simulink model "waterTankBurner"  (R2014b)
settings: Solver=ode1  StartTime=0.0  StopTime=100  FixedStep=0.0001  MaxStep=0.0001  RelTol=1e-3
(part 2 of 4)

== system waterTankBurner/waterTank31 ==
  note: integrator t4
  ON : Inport
  OFF : Inport  Port=2
  INIT y1 : Constant  Value=20
  INIT y3 : Constant  Value=100
  Integrator b{1..4} (4 alike) : DiscreteIntegrator  ExternalReset=either  InitialConditionSource=external  InitialCondition=510  InitialConditionSetting=State (most efficient)  SampleTime=-1
  MATLAB Function : MATLAB Function  Priority=1  TreatAsAtomicUnit=on
  MATLAB Function1 : MATLAB Function  TreatAsAtomicUnit=on
  Multiport Switch : MultiPortSwitch  Inputs=4
  Scope : Scope  NumInputPorts=8
      settings: TickLabels=on  ShowLegends=on  YMin=0~0~0~0~0~0~0~0  YMax=1~1~1~1~1~1~1~1
  q : Memory  X0=1  LinearizeMemory=on
  reset1 : Memory  LinearizeMemory=on
  xx : Memory  LinearizeMemory=on
  x : Outport
  wires:
  INIT y1/1 -> Integrator b1/3
  MATLAB Function1/1(ode1) -> Integrator b1/1
  MATLAB Function/1(qNext) -> q/1  "q_before"
  q/1 -> Multiport Switch/1, MATLAB Function/1(q), Scope/1  "q_after"
  MATLAB Function/2(reset) -> reset1/1
  MATLAB Function1/2(ode2) -> Integrator b2/1
  INIT y3/1 -> Integrator b3/3
  MATLAB Function1/3(ode3) -> Integrator b3/1
  MATLAB Function1/4(ode4) -> Integrator b4/1
  reset1/1 -> Integrator b4/2, Integrator b3/2, Integrator b2/2, Integrator b1/2  "reset_after"
  Integrator b1/1 -> Multiport Switch/2  "integrator t1"
  Integrator b2/1 -> Multiport Switch/3  "integrator t2"
  Integrator b3/1 -> Multiport Switch/4  "integrator t3"
  Integrator b4/1 -> Multiport Switch/5
  OFF/1 -> MATLAB Function/3(OFF)
  ON/1 -> MATLAB Function/2(ON)
  xx/1 -> x/1, Scope/2, Integrator b2/3, Integrator b4/3, MATLAB Function1/1(x), MATLAB Function/4(x)
  Multiport Switch/1 -> xx/1  "x"

== system waterTankBurner/waterTank32 ==
  note: integrator t4
  ON : Inport
  OFF : Inport  Port=2
  INIT y1 : Constant  Value=20
  INIT y3 : Constant  Value=100
  Integrator b{1..4} (4 alike) : DiscreteIntegrator  ExternalReset=either  InitialConditionSource=external  InitialCondition=510  InitialConditionSetting=State (most efficient)  SampleTime=-1
  MATLAB Function : MATLAB Function  Priority=1  TreatAsAtomicUnit=on
  MATLAB Function1 : MATLAB Function  TreatAsAtomicUnit=on
  Multiport Switch : MultiPortSwitch  Inputs=4
  Scope : Scope  NumInputPorts=8
      settings: TickLabels=on  ShowLegends=on  YMin=0~0~0~0~0~0~0~0  YMax=1~1~1~1~1~1~1~1
  q : Memory  X0=1  LinearizeMemory=on
  reset1 : Memory  LinearizeMemory=on
  xx : Memory  LinearizeMemory=on
  x : Outport
  wires:
  INIT y1/1 -> Integrator b1/3
  MATLAB Function1/1(ode1) -> Integrator b1/1
  MATLAB Function/1(qNext) -> q/1  "q_before"
  q/1 -> Multiport Switch/1, MATLAB Function/1(q), Scope/1  "q_after"
  MATLAB Function/2(reset) -> reset1/1
  MATLAB Function1/2(ode2) -> Integrator b2/1
  INIT y3/1 -> Integrator b3/3
  MATLAB Function1/3(ode3) -> Integrator b3/1
  MATLAB Function1/4(ode4) -> Integrator b4/1
  reset1/1 -> Integrator b4/2, Integrator b3/2, Integrator b2/2, Integrator b1/2  "reset_after"
  Integrator b1/1 -> Multiport Switch/2  "integrator t1"
  Integrator b2/1 -> Multiport Switch/3  "integrator t2"
  Integrator b3/1 -> Multiport Switch/4  "integrator t3"
  Integrator b4/1 -> Multiport Switch/5
  OFF/1 -> MATLAB Function/3(OFF)
  ON/1 -> MATLAB Function/2(ON)
  xx/1 -> x/1, Scope/2, Integrator b2/3, Integrator b4/3, MATLAB Function1/1(x), MATLAB Function/4(x)
  Multiport Switch/1 -> xx/1  "x"

== system waterTankBurner/waterTank33 ==
  note: integrator t4
  ON : Inport
  OFF : Inport  Port=2
  INIT y1 : Constant  Value=20
  INIT y3 : Constant  Value=100
  Integrator b{1..4} (4 alike) : DiscreteIntegrator  ExternalReset=either  InitialConditionSource=external  InitialCondition=510  InitialConditionSetting=State (most efficient)  SampleTime=-1
  MATLAB Function : MATLAB Function  Priority=1  TreatAsAtomicUnit=on
  MATLAB Function1 : MATLAB Function  TreatAsAtomicUnit=on
  Multiport Switch : MultiPortSwitch  Inputs=4
  Scope : Scope  NumInputPorts=8
      settings: TickLabels=on  ShowLegends=on  YMin=0~0~0~0~0~0~0~0  YMax=1~1~1~1~1~1~1~1
  q : Memory  X0=1  LinearizeMemory=on
  reset1 : Memory  LinearizeMemory=on
  xx : Memory  LinearizeMemory=on
  x : Outport
  wires:
  INIT y1/1 -> Integrator b1/3
  MATLAB Function1/1(ode1) -> Integrator b1/1
  MATLAB Function/1(qNext) -> q/1  "q_before"
  q/1 -> Multiport Switch/1, MATLAB Function/1(q), Scope/1  "q_after"
  MATLAB Function/2(reset) -> reset1/1
  MATLAB Function1/2(ode2) -> Integrator b2/1
  INIT y3/1 -> Integrator b3/3
  MATLAB Function1/3(ode3) -> Integrator b3/1
  MATLAB Function1/4(ode4) -> Integrator b4/1
  reset1/1 -> Integrator b4/2, Integrator b3/2, Integrator b2/2, Integrator b1/2  "reset_after"
  Integrator b1/1 -> Multiport Switch/2  "integrator t1"
  Integrator b2/1 -> Multiport Switch/3  "integrator t2"
  Integrator b3/1 -> Multiport Switch/4  "integrator t3"
  Integrator b4/1 -> Multiport Switch/5
  OFF/1 -> MATLAB Function/3(OFF)
  ON/1 -> MATLAB Function/2(ON)
  xx/1 -> x/1, Scope/2, Integrator b2/3, Integrator b4/3, MATLAB Function1/1(x), MATLAB Function/4(x)
  Multiport Switch/1 -> xx/1  "x"

== system waterTankBurner/waterTank34 ==
  note: integrator t4
  ON : Inport
  OFF : Inport  Port=2
  INIT y1 : Constant  Value=20
  INIT y3 : Constant  Value=100
  Integrator b{1..4} (4 alike) : DiscreteIntegrator  ExternalReset=either  InitialConditionSource=external  InitialCondition=510  InitialConditionSetting=State (most efficient)  SampleTime=-1
  MATLAB Function : MATLAB Function  Priority=1  TreatAsAtomicUnit=on
  MATLAB Function1 : MATLAB Function  TreatAsAtomicUnit=on
  Multiport Switch : MultiPortSwitch  Inputs=4
  Scope : Scope  NumInputPorts=8
      settings: TickLabels=on  ShowLegends=on  YMin=0~0~0~0~0~0~0~0  YMax=1~1~1~1~1~1~1~1
  q : Memory  X0=1  LinearizeMemory=on
  reset1 : Memory  LinearizeMemory=on
  xx : Memory  LinearizeMemory=on
  x : Outport
  wires:
  INIT y1/1 -> Integrator b1/3
  MATLAB Function1/1(ode1) -> Integrator b1/1
  MATLAB Function/1(qNext) -> q/1  "q_before"
  q/1 -> Multiport Switch/1, MATLAB Function/1(q), Scope/1  "q_after"
  MATLAB Function/2(reset) -> reset1/1
  MATLAB Function1/2(ode2) -> Integrator b2/1
  INIT y3/1 -> Integrator b3/3
  MATLAB Function1/3(ode3) -> Integrator b3/1
  MATLAB Function1/4(ode4) -> Integrator b4/1
  reset1/1 -> Integrator b4/2, Integrator b3/2, Integrator b2/2, Integrator b1/2  "reset_after"
  Integrator b1/1 -> Multiport Switch/2  "integrator t1"
  Integrator b2/1 -> Multiport Switch/3  "integrator t2"
  Integrator b3/1 -> Multiport Switch/4  "integrator t3"
  Integrator b4/1 -> Multiport Switch/5
  OFF/1 -> MATLAB Function/3(OFF)
  ON/1 -> MATLAB Function/2(ON)
  xx/1 -> x/1, Scope/2, Integrator b2/3, Integrator b4/3, MATLAB Function1/1(x), MATLAB Function/4(x)
  Multiport Switch/1 -> xx/1  "x"

== system waterTankBurner/waterTank35 ==
  note: integrator t4
  ON : Inport
  OFF : Inport  Port=2
  INIT y1 : Constant  Value=20
  INIT y3 : Constant  Value=100
  Integrator b{1..4} (4 alike) : DiscreteIntegrator  ExternalReset=either  InitialConditionSource=external  InitialCondition=510  InitialConditionSetting=State (most efficient)  SampleTime=-1
  MATLAB Function : MATLAB Function  Priority=1  TreatAsAtomicUnit=on
  MATLAB Function1 : MATLAB Function  TreatAsAtomicUnit=on
  Multiport Switch : MultiPortSwitch  Inputs=4
  Scope : Scope  NumInputPorts=8
      settings: TickLabels=on  ShowLegends=on  YMin=0~0~0~0~0~0~0~0  YMax=1~1~1~1~1~1~1~1
  q : Memory  X0=1  LinearizeMemory=on
  reset1 : Memory  LinearizeMemory=on
  xx : Memory  LinearizeMemory=on
  x : Outport
  wires:
  INIT y1/1 -> Integrator b1/3
  MATLAB Function1/1(ode1) -> Integrator b1/1
  MATLAB Function/1(qNext) -> q/1  "q_before"
  q/1 -> Multiport Switch/1, MATLAB Function/1(q), Scope/1  "q_after"
  MATLAB Function/2(reset) -> reset1/1
  MATLAB Function1/2(ode2) -> Integrator b2/1
  INIT y3/1 -> Integrator b3/3
  MATLAB Function1/3(ode3) -> Integrator b3/1
  MATLAB Function1/4(ode4) -> Integrator b4/1
  reset1/1 -> Integrator b4/2, Integrator b3/2, Integrator b2/2, Integrator b1/2  "reset_after"
  Integrator b1/1 -> Multiport Switch/2  "integrator t1"
  Integrator b2/1 -> Multiport Switch/3  "integrator t2"
  Integrator b3/1 -> Multiport Switch/4  "integrator t3"
  Integrator b4/1 -> Multiport Switch/5
  OFF/1 -> MATLAB Function/3(OFF)
  ON/1 -> MATLAB Function/2(ON)
  xx/1 -> x/1, Scope/2, Integrator b2/3, Integrator b4/3, MATLAB Function1/1(x), MATLAB Function/4(x)
  Multiport Switch/1 -> xx/1  "x"

== system waterTankBurner/waterTank36 ==
  note: integrator t4
  ON : Inport
  OFF : Inport  Port=2
  INIT y1 : Constant  Value=20
  INIT y3 : Constant  Value=100
  Integrator b{1..4} (4 alike) : DiscreteIntegrator  ExternalReset=either  InitialConditionSource=external  InitialCondition=510  InitialConditionSetting=State (most efficient)  SampleTime=-1
  MATLAB Function : MATLAB Function  Priority=1  TreatAsAtomicUnit=on
  MATLAB Function1 : MATLAB Function  TreatAsAtomicUnit=on
  Multiport Switch : MultiPortSwitch  Inputs=4
  Scope : Scope  NumInputPorts=8
      settings: TickLabels=on  ShowLegends=on  YMin=0~0~0~0~0~0~0~0  YMax=1~1~1~1~1~1~1~1
  q : Memory  X0=1  LinearizeMemory=on
  reset1 : Memory  LinearizeMemory=on
  xx : Memory  LinearizeMemory=on
  x : Outport
  wires:
  INIT y1/1 -> Integrator b1/3
  MATLAB Function1/1(ode1) -> Integrator b1/1
  MATLAB Function/1(qNext) -> q/1  "q_before"
  q/1 -> Multiport Switch/1, MATLAB Function/1(q), Scope/1  "q_after"
  MATLAB Function/2(reset) -> reset1/1
  MATLAB Function1/2(ode2) -> Integrator b2/1
  INIT y3/1 -> Integrator b3/3
  MATLAB Function1/3(ode3) -> Integrator b3/1
  MATLAB Function1/4(ode4) -> Integrator b4/1
  reset1/1 -> Integrator b4/2, Integrator b3/2, Integrator b2/2, Integrator b1/2  "reset_after"
  Integrator b1/1 -> Multiport Switch/2  "integrator t1"
  Integrator b2/1 -> Multiport Switch/3  "integrator t2"
  Integrator b3/1 -> Multiport Switch/4  "integrator t3"
  Integrator b4/1 -> Multiport Switch/5
  OFF/1 -> MATLAB Function/3(OFF)
  ON/1 -> MATLAB Function/2(ON)
  xx/1 -> x/1, Scope/2, Integrator b2/3, Integrator b4/3, MATLAB Function1/1(x), MATLAB Function/4(x)
  Multiport Switch/1 -> xx/1  "x"

== system waterTankBurner/waterTank37 ==
  note: integrator t4
  ON : Inport
  OFF : Inport  Port=2
  INIT y1 : Constant  Value=20
  INIT y3 : Constant  Value=100
  Integrator b{1..4} (4 alike) : DiscreteIntegrator  ExternalReset=either  InitialConditionSource=external  InitialCondition=510  InitialConditionSetting=State (most efficient)  SampleTime=-1
  MATLAB Function : MATLAB Function  Priority=1  TreatAsAtomicUnit=on
  MATLAB Function1 : MATLAB Function  TreatAsAtomicUnit=on
  Multiport Switch : MultiPortSwitch  Inputs=4
  Scope : Scope  NumInputPorts=8
      settings: TickLabels=on  ShowLegends=on  YMin=0~0~0~0~0~0~0~0  YMax=1~1~1~1~1~1~1~1
  q : Memory  X0=1  LinearizeMemory=on
  reset1 : Memory  LinearizeMemory=on
  xx : Memory  LinearizeMemory=on
  x : Outport
  wires:
  INIT y1/1 -> Integrator b1/3
  MATLAB Function1/1(ode1) -> Integrator b1/1
  MATLAB Function/1(qNext) -> q/1  "q_before"
  q/1 -> Multiport Switch/1, MATLAB Function/1(q), Scope/1  "q_after"
  MATLAB Function/2(reset) -> reset1/1
  MATLAB Function1/2(ode2) -> Integrator b2/1
  INIT y3/1 -> Integrator b3/3
  MATLAB Function1/3(ode3) -> Integrator b3/1
  MATLAB Function1/4(ode4) -> Integrator b4/1
  reset1/1 -> Integrator b4/2, Integrator b3/2, Integrator b2/2, Integrator b1/2  "reset_after"
  Integrator b1/1 -> Multiport Switch/2  "integrator t1"
  Integrator b2/1 -> Multiport Switch/3  "integrator t2"
  Integrator b3/1 -> Multiport Switch/4  "integrator t3"
  Integrator b4/1 -> Multiport Switch/5
  OFF/1 -> MATLAB Function/3(OFF)
  ON/1 -> MATLAB Function/2(ON)
  xx/1 -> x/1, Scope/2, Integrator b2/3, Integrator b4/3, MATLAB Function1/1(x), MATLAB Function/4(x)
  Multiport Switch/1 -> xx/1  "x"

== system waterTankBurner/waterTank38 ==
  note: integrator t4
  ON : Inport
  OFF : Inport  Port=2
  INIT y1 : Constant  Value=20
  INIT y3 : Constant  Value=100
  Integrator b{1..4} (4 alike) : DiscreteIntegrator  ExternalReset=either  InitialConditionSource=external  InitialCondition=510  InitialConditionSetting=State (most efficient)  SampleTime=-1
  MATLAB Function : MATLAB Function  Priority=1  TreatAsAtomicUnit=on
  MATLAB Function1 : MATLAB Function  TreatAsAtomicUnit=on
  Multiport Switch : MultiPortSwitch  Inputs=4
  Scope : Scope  NumInputPorts=8
      settings: TickLabels=on  ShowLegends=on  YMin=0~0~0~0~0~0~0~0  YMax=1~1~1~1~1~1~1~1
  q : Memory  X0=1  LinearizeMemory=on
  reset1 : Memory  LinearizeMemory=on
  xx : Memory  LinearizeMemory=on
  x : Outport
  wires:
  INIT y1/1 -> Integrator b1/3
  MATLAB Function1/1(ode1) -> Integrator b1/1
  MATLAB Function/1(qNext) -> q/1  "q_before"
  q/1 -> Multiport Switch/1, MATLAB Function/1(q), Scope/1  "q_after"
  MATLAB Function/2(reset) -> reset1/1
  MATLAB Function1/2(ode2) -> Integrator b2/1
  INIT y3/1 -> Integrator b3/3
  MATLAB Function1/3(ode3) -> Integrator b3/1
  MATLAB Function1/4(ode4) -> Integrator b4/1
  reset1/1 -> Integrator b4/2, Integrator b3/2, Integrator b2/2, Integrator b1/2  "reset_after"
  Integrator b1/1 -> Multiport Switch/2  "integrator t1"
  Integrator b2/1 -> Multiport Switch/3  "integrator t2"
  Integrator b3/1 -> Multiport Switch/4  "integrator t3"
  Integrator b4/1 -> Multiport Switch/5
  OFF/1 -> MATLAB Function/3(OFF)
  ON/1 -> MATLAB Function/2(ON)
  xx/1 -> x/1, Scope/2, Integrator b2/3, Integrator b4/3, MATLAB Function1/1(x), MATLAB Function/4(x)
  Multiport Switch/1 -> xx/1  "x"

== system waterTankBurner/waterTank39 ==
  note: integrator t4
  ON : Inport
  OFF : Inport  Port=2
  INIT y1 : Constant  Value=20
  INIT y3 : Constant  Value=100
  Integrator b{1..4} (4 alike) : DiscreteIntegrator  ExternalReset=either  InitialConditionSource=external  InitialCondition=510  InitialConditionSetting=State (most efficient)  SampleTime=-1
  MATLAB Function : MATLAB Function  Priority=1  TreatAsAtomicUnit=on
  MATLAB Function1 : MATLAB Function  TreatAsAtomicUnit=on
  Multiport Switch : MultiPortSwitch  Inputs=4
  Scope : Scope  NumInputPorts=8
      settings: TickLabels=on  ShowLegends=on  YMin=0~0~0~0~0~0~0~0  YMax=1~1~1~1~1~1~1~1
  q : Memory  X0=1  LinearizeMemory=on
  reset1 : Memory  LinearizeMemory=on
  xx : Memory  LinearizeMemory=on
  x : Outport
  wires:
  INIT y1/1 -> Integrator b1/3
  MATLAB Function1/1(ode1) -> Integrator b1/1
  MATLAB Function/1(qNext) -> q/1  "q_before"
  q/1 -> Multiport Switch/1, MATLAB Function/1(q), Scope/1  "q_after"
  MATLAB Function/2(reset) -> reset1/1
  MATLAB Function1/2(ode2) -> Integrator b2/1
  INIT y3/1 -> Integrator b3/3
  MATLAB Function1/3(ode3) -> Integrator b3/1
  MATLAB Function1/4(ode4) -> Integrator b4/1
  reset1/1 -> Integrator b4/2, Integrator b3/2, Integrator b2/2, Integrator b1/2  "reset_after"
  Integrator b1/1 -> Multiport Switch/2  "integrator t1"
  Integrator b2/1 -> Multiport Switch/3  "integrator t2"
  Integrator b3/1 -> Multiport Switch/4  "integrator t3"
  Integrator b4/1 -> Multiport Switch/5
  OFF/1 -> MATLAB Function/3(OFF)
  ON/1 -> MATLAB Function/2(ON)
  xx/1 -> x/1, Scope/2, Integrator b2/3, Integrator b4/3, MATLAB Function1/1(x), MATLAB Function/4(x)
  Multiport Switch/1 -> xx/1  "x"

== system waterTankBurner/waterTank4 ==
  note: integrator t4
  ON : Inport
  OFF : Inport  Port=2
  INIT y1 : Constant  Value=20
  INIT y3 : Constant  Value=100
  Integrator b{1..4} (4 alike) : DiscreteIntegrator  ExternalReset=either  InitialConditionSource=external  InitialCondition=510  InitialConditionSetting=State (most efficient)  SampleTime=-1
  MATLAB Function : MATLAB Function  Priority=1  TreatAsAtomicUnit=on
  MATLAB Function1 : MATLAB Function  TreatAsAtomicUnit=on
  Multiport Switch : MultiPortSwitch  Inputs=4
  Scope : Scope  NumInputPorts=8
      settings: TickLabels=on  ShowLegends=on  YMin=0~0~0~0~0~0~0~0  YMax=1~1~1~1~1~1~1~1
  q : Memory  X0=1  LinearizeMemory=on
  reset1 : Memory  LinearizeMemory=on
  xx : Memory  LinearizeMemory=on
  x : Outport
  wires:
  INIT y1/1 -> Integrator b1/3
  MATLAB Function1/1(ode1) -> Integrator b1/1
  MATLAB Function/1(qNext) -> q/1  "q_before"
  q/1 -> Multiport Switch/1, MATLAB Function/1(q), Scope/1  "q_after"
  MATLAB Function/2(reset) -> reset1/1
  MATLAB Function1/2(ode2) -> Integrator b2/1
  INIT y3/1 -> Integrator b3/3
  MATLAB Function1/3(ode3) -> Integrator b3/1
  MATLAB Function1/4(ode4) -> Integrator b4/1
  reset1/1 -> Integrator b4/2, Integrator b3/2, Integrator b2/2, Integrator b1/2  "reset_after"
  Integrator b1/1 -> Multiport Switch/2  "integrator t1"
  Integrator b2/1 -> Multiport Switch/3  "integrator t2"
  Integrator b3/1 -> Multiport Switch/4  "integrator t3"
  Integrator b4/1 -> Multiport Switch/5
  OFF/1 -> MATLAB Function/3(OFF)
  ON/1 -> MATLAB Function/2(ON)
  xx/1 -> x/1, Scope/2, Integrator b2/3, Integrator b4/3, MATLAB Function1/1(x), MATLAB Function/4(x)
  Multiport Switch/1 -> xx/1  "x"

== system waterTankBurner/waterTank40 ==
  note: integrator t4
  ON : Inport
  OFF : Inport  Port=2
  INIT y1 : Constant  Value=20
  INIT y3 : Constant  Value=100
  Integrator b{1..4} (4 alike) : DiscreteIntegrator  ExternalReset=either  InitialConditionSource=external  InitialCondition=510  InitialConditionSetting=State (most efficient)  SampleTime=-1
  MATLAB Function : MATLAB Function  Priority=1  TreatAsAtomicUnit=on
  MATLAB Function1 : MATLAB Function  TreatAsAtomicUnit=on
  Multiport Switch : MultiPortSwitch  Inputs=4
  Scope : Scope  NumInputPorts=8
      settings: TickLabels=on  ShowLegends=on  YMin=0~0~0~0~0~0~0~0  YMax=1~1~1~1~1~1~1~1
  q : Memory  X0=1  LinearizeMemory=on
  reset1 : Memory  LinearizeMemory=on
  xx : Memory  LinearizeMemory=on
  x : Outport
  wires:
  INIT y1/1 -> Integrator b1/3
  MATLAB Function1/1(ode1) -> Integrator b1/1
  MATLAB Function/1(qNext) -> q/1  "q_before"
  q/1 -> Multiport Switch/1, MATLAB Function/1(q), Scope/1  "q_after"
  MATLAB Function/2(reset) -> reset1/1
  MATLAB Function1/2(ode2) -> Integrator b2/1
  INIT y3/1 -> Integrator b3/3
  MATLAB Function1/3(ode3) -> Integrator b3/1
  MATLAB Function1/4(ode4) -> Integrator b4/1
  reset1/1 -> Integrator b4/2, Integrator b3/2, Integrator b2/2, Integrator b1/2  "reset_after"
  Integrator b1/1 -> Multiport Switch/2  "integrator t1"
  Integrator b2/1 -> Multiport Switch/3  "integrator t2"
  Integrator b3/1 -> Multiport Switch/4  "integrator t3"
  Integrator b4/1 -> Multiport Switch/5
  OFF/1 -> MATLAB Function/3(OFF)
  ON/1 -> MATLAB Function/2(ON)
  xx/1 -> x/1, Scope/2, Integrator b2/3, Integrator b4/3, MATLAB Function1/1(x), MATLAB Function/4(x)
  Multiport Switch/1 -> xx/1  "x"

== system waterTankBurner/waterTank41 ==
  note: integrator t4
  ON : Inport
  OFF : Inport  Port=2
  INIT y1 : Constant  Value=20
  INIT y3 : Constant  Value=100
  Integrator b{1..4} (4 alike) : DiscreteIntegrator  ExternalReset=either  InitialConditionSource=external  InitialCondition=510  InitialConditionSetting=State (most efficient)  SampleTime=-1
  MATLAB Function : MATLAB Function  Priority=1  TreatAsAtomicUnit=on
  MATLAB Function1 : MATLAB Function  TreatAsAtomicUnit=on
  Multiport Switch : MultiPortSwitch  Inputs=4
  Scope : Scope  NumInputPorts=8
      settings: TickLabels=on  ShowLegends=on  YMin=0~0~0~0~0~0~0~0  YMax=1~1~1~1~1~1~1~1
  q : Memory  X0=1  LinearizeMemory=on
  reset1 : Memory  LinearizeMemory=on
  xx : Memory  LinearizeMemory=on
  x : Outport
  wires:
  INIT y1/1 -> Integrator b1/3
  MATLAB Function1/1(ode1) -> Integrator b1/1
  MATLAB Function/1(qNext) -> q/1  "q_before"
  q/1 -> Multiport Switch/1, MATLAB Function/1(q), Scope/1  "q_after"
  MATLAB Function/2(reset) -> reset1/1
  MATLAB Function1/2(ode2) -> Integrator b2/1
  INIT y3/1 -> Integrator b3/3
  MATLAB Function1/3(ode3) -> Integrator b3/1
  MATLAB Function1/4(ode4) -> Integrator b4/1
  reset1/1 -> Integrator b4/2, Integrator b3/2, Integrator b2/2, Integrator b1/2  "reset_after"
  Integrator b1/1 -> Multiport Switch/2  "integrator t1"
  Integrator b2/1 -> Multiport Switch/3  "integrator t2"
  Integrator b3/1 -> Multiport Switch/4  "integrator t3"
  Integrator b4/1 -> Multiport Switch/5
  OFF/1 -> MATLAB Function/3(OFF)
  ON/1 -> MATLAB Function/2(ON)
  xx/1 -> x/1, Scope/2, Integrator b2/3, Integrator b4/3, MATLAB Function1/1(x), MATLAB Function/4(x)
  Multiport Switch/1 -> xx/1  "x"

== system waterTankBurner/waterTank42 ==
  note: integrator t4
  ON : Inport
  OFF : Inport  Port=2
  INIT y1 : Constant  Value=20
  INIT y3 : Constant  Value=100
  Integrator b{1..4} (4 alike) : DiscreteIntegrator  ExternalReset=either  InitialConditionSource=external  InitialCondition=510  InitialConditionSetting=State (most efficient)  SampleTime=-1
  MATLAB Function : MATLAB Function  Priority=1  TreatAsAtomicUnit=on
  MATLAB Function1 : MATLAB Function  TreatAsAtomicUnit=on
  Multiport Switch : MultiPortSwitch  Inputs=4
  Scope : Scope  NumInputPorts=8
      settings: TickLabels=on  ShowLegends=on  YMin=0~0~0~0~0~0~0~0  YMax=1~1~1~1~1~1~1~1
  q : Memory  X0=1  LinearizeMemory=on
  reset1 : Memory  LinearizeMemory=on
  xx : Memory  LinearizeMemory=on
  x : Outport
  wires:
  INIT y1/1 -> Integrator b1/3
  MATLAB Function1/1(ode1) -> Integrator b1/1
  MATLAB Function/1(qNext) -> q/1  "q_before"
  q/1 -> Multiport Switch/1, MATLAB Function/1(q), Scope/1  "q_after"
  MATLAB Function/2(reset) -> reset1/1
  MATLAB Function1/2(ode2) -> Integrator b2/1
  INIT y3/1 -> Integrator b3/3
  MATLAB Function1/3(ode3) -> Integrator b3/1
  MATLAB Function1/4(ode4) -> Integrator b4/1
  reset1/1 -> Integrator b4/2, Integrator b3/2, Integrator b2/2, Integrator b1/2  "reset_after"
  Integrator b1/1 -> Multiport Switch/2  "integrator t1"
  Integrator b2/1 -> Multiport Switch/3  "integrator t2"
  Integrator b3/1 -> Multiport Switch/4  "integrator t3"
  Integrator b4/1 -> Multiport Switch/5
  OFF/1 -> MATLAB Function/3(OFF)
  ON/1 -> MATLAB Function/2(ON)
  xx/1 -> x/1, Scope/2, Integrator b2/3, Integrator b4/3, MATLAB Function1/1(x), MATLAB Function/4(x)
  Multiport Switch/1 -> xx/1  "x"

== system waterTankBurner/waterTank43 ==
  note: integrator t4
  ON : Inport
  OFF : Inport  Port=2
  INIT y1 : Constant  Value=20
  INIT y3 : Constant  Value=100
  Integrator b{1..4} (4 alike) : DiscreteIntegrator  ExternalReset=either  InitialConditionSource=external  InitialCondition=510  InitialConditionSetting=State (most efficient)  SampleTime=-1
  MATLAB Function : MATLAB Function  Priority=1  TreatAsAtomicUnit=on
  MATLAB Function1 : MATLAB Function  TreatAsAtomicUnit=on
  Multiport Switch : MultiPortSwitch  Inputs=4
  Scope : Scope  NumInputPorts=8
      settings: TickLabels=on  ShowLegends=on  YMin=0~0~0~0~0~0~0~0  YMax=1~1~1~1~1~1~1~1
  q : Memory  X0=1  LinearizeMemory=on
  reset1 : Memory  LinearizeMemory=on
  xx : Memory  LinearizeMemory=on
  x : Outport
  wires:
  INIT y1/1 -> Integrator b1/3
  MATLAB Function1/1(ode1) -> Integrator b1/1
  MATLAB Function/1(qNext) -> q/1  "q_before"
  q/1 -> Multiport Switch/1, MATLAB Function/1(q), Scope/1  "q_after"
  MATLAB Function/2(reset) -> reset1/1
  MATLAB Function1/2(ode2) -> Integrator b2/1
  INIT y3/1 -> Integrator b3/3
  MATLAB Function1/3(ode3) -> Integrator b3/1
  MATLAB Function1/4(ode4) -> Integrator b4/1
  reset1/1 -> Integrator b4/2, Integrator b3/2, Integrator b2/2, Integrator b1/2  "reset_after"
  Integrator b1/1 -> Multiport Switch/2  "integrator t1"
  Integrator b2/1 -> Multiport Switch/3  "integrator t2"
  Integrator b3/1 -> Multiport Switch/4  "integrator t3"
  Integrator b4/1 -> Multiport Switch/5
  OFF/1 -> MATLAB Function/3(OFF)
  ON/1 -> MATLAB Function/2(ON)
  xx/1 -> x/1, Scope/2, Integrator b2/3, Integrator b4/3, MATLAB Function1/1(x), MATLAB Function/4(x)
  Multiport Switch/1 -> xx/1  "x"

== system waterTankBurner/waterTank44 ==
  note: integrator t4
  ON : Inport
  OFF : Inport  Port=2
  INIT y1 : Constant  Value=20
  INIT y3 : Constant  Value=100
  Integrator b{1..4} (4 alike) : DiscreteIntegrator  ExternalReset=either  InitialConditionSource=external  InitialCondition=510  InitialConditionSetting=State (most efficient)  SampleTime=-1
  MATLAB Function : MATLAB Function  Priority=1  TreatAsAtomicUnit=on
  MATLAB Function1 : MATLAB Function  TreatAsAtomicUnit=on
  Multiport Switch : MultiPortSwitch  Inputs=4
  Scope : Scope  NumInputPorts=8
      settings: TickLabels=on  ShowLegends=on  YMin=0~0~0~0~0~0~0~0  YMax=1~1~1~1~1~1~1~1
  q : Memory  X0=1  LinearizeMemory=on
  reset1 : Memory  LinearizeMemory=on
  xx : Memory  LinearizeMemory=on
  x : Outport
  wires:
  INIT y1/1 -> Integrator b1/3
  MATLAB Function1/1(ode1) -> Integrator b1/1
  MATLAB Function/1(qNext) -> q/1  "q_before"
  q/1 -> Multiport Switch/1, MATLAB Function/1(q), Scope/1  "q_after"
  MATLAB Function/2(reset) -> reset1/1
  MATLAB Function1/2(ode2) -> Integrator b2/1
  INIT y3/1 -> Integrator b3/3
  MATLAB Function1/3(ode3) -> Integrator b3/1
  MATLAB Function1/4(ode4) -> Integrator b4/1
  reset1/1 -> Integrator b4/2, Integrator b3/2, Integrator b2/2, Integrator b1/2  "reset_after"
  Integrator b1/1 -> Multiport Switch/2  "integrator t1"
  Integrator b2/1 -> Multiport Switch/3  "integrator t2"
  Integrator b3/1 -> Multiport Switch/4  "integrator t3"
  Integrator b4/1 -> Multiport Switch/5
  OFF/1 -> MATLAB Function/3(OFF)
  ON/1 -> MATLAB Function/2(ON)
  xx/1 -> x/1, Scope/2, Integrator b2/3, Integrator b4/3, MATLAB Function1/1(x), MATLAB Function/4(x)
  Multiport Switch/1 -> xx/1  "x"

== system waterTankBurner/waterTank45 ==
  note: integrator t4
  ON : Inport
  OFF : Inport  Port=2
  INIT y1 : Constant  Value=20
  INIT y3 : Constant  Value=100
  Integrator b{1..4} (4 alike) : DiscreteIntegrator  ExternalReset=either  InitialConditionSource=external  InitialCondition=510  InitialConditionSetting=State (most efficient)  SampleTime=-1
  MATLAB Function : MATLAB Function  Priority=1  TreatAsAtomicUnit=on
  MATLAB Function1 : MATLAB Function  TreatAsAtomicUnit=on
  Multiport Switch : MultiPortSwitch  Inputs=4
  Scope : Scope  NumInputPorts=8
      settings: TickLabels=on  ShowLegends=on  YMin=0~0~0~0~0~0~0~0  YMax=1~1~1~1~1~1~1~1
  q : Memory  X0=1  LinearizeMemory=on
  reset1 : Memory  LinearizeMemory=on
  xx : Memory  LinearizeMemory=on
  x : Outport
  wires:
  INIT y1/1 -> Integrator b1/3
  MATLAB Function1/1(ode1) -> Integrator b1/1
  MATLAB Function/1(qNext) -> q/1  "q_before"
  q/1 -> Multiport Switch/1, MATLAB Function/1(q), Scope/1  "q_after"
  MATLAB Function/2(reset) -> reset1/1
  MATLAB Function1/2(ode2) -> Integrator b2/1
  INIT y3/1 -> Integrator b3/3
  MATLAB Function1/3(ode3) -> Integrator b3/1
  MATLAB Function1/4(ode4) -> Integrator b4/1
  reset1/1 -> Integrator b4/2, Integrator b3/2, Integrator b2/2, Integrator b1/2  "reset_after"
  Integrator b1/1 -> Multiport Switch/2  "integrator t1"
  Integrator b2/1 -> Multiport Switch/3  "integrator t2"
  Integrator b3/1 -> Multiport Switch/4  "integrator t3"
  Integrator b4/1 -> Multiport Switch/5
  OFF/1 -> MATLAB Function/3(OFF)
  ON/1 -> MATLAB Function/2(ON)
  xx/1 -> x/1, Scope/2, Integrator b2/3, Integrator b4/3, MATLAB Function1/1(x), MATLAB Function/4(x)
  Multiport Switch/1 -> xx/1  "x"

== system waterTankBurner/waterTank46 ==
  note: integrator t4
  ON : Inport
  OFF : Inport  Port=2
  INIT y1 : Constant  Value=20
  INIT y3 : Constant  Value=100
  Integrator b{1..4} (4 alike) : DiscreteIntegrator  ExternalReset=either  InitialConditionSource=external  InitialCondition=510  InitialConditionSetting=State (most efficient)  SampleTime=-1
  MATLAB Function : MATLAB Function  Priority=1  TreatAsAtomicUnit=on
  MATLAB Function1 : MATLAB Function  TreatAsAtomicUnit=on
  Multiport Switch : MultiPortSwitch  Inputs=4
  Scope : Scope  NumInputPorts=8
      settings: TickLabels=on  ShowLegends=on  YMin=0~0~0~0~0~0~0~0  YMax=1~1~1~1~1~1~1~1
  q : Memory  X0=1  LinearizeMemory=on
  reset1 : Memory  LinearizeMemory=on
  xx : Memory  LinearizeMemory=on
  x : Outport
  wires:
  INIT y1/1 -> Integrator b1/3
  MATLAB Function1/1(ode1) -> Integrator b1/1
  MATLAB Function/1(qNext) -> q/1  "q_before"
  q/1 -> Multiport Switch/1, MATLAB Function/1(q), Scope/1  "q_after"
  MATLAB Function/2(reset) -> reset1/1
  MATLAB Function1/2(ode2) -> Integrator b2/1
  INIT y3/1 -> Integrator b3/3
  MATLAB Function1/3(ode3) -> Integrator b3/1
  MATLAB Function1/4(ode4) -> Integrator b4/1
  reset1/1 -> Integrator b4/2, Integrator b3/2, Integrator b2/2, Integrator b1/2  "reset_after"
  Integrator b1/1 -> Multiport Switch/2  "integrator t1"
  Integrator b2/1 -> Multiport Switch/3  "integrator t2"
  Integrator b3/1 -> Multiport Switch/4  "integrator t3"
  Integrator b4/1 -> Multiport Switch/5
  OFF/1 -> MATLAB Function/3(OFF)
  ON/1 -> MATLAB Function/2(ON)
  xx/1 -> x/1, Scope/2, Integrator b2/3, Integrator b4/3, MATLAB Function1/1(x), MATLAB Function/4(x)
  Multiport Switch/1 -> xx/1  "x"

== system waterTankBurner/waterTank47 ==
  note: integrator t4
  ON : Inport
  OFF : Inport  Port=2
  INIT y1 : Constant  Value=20
  INIT y3 : Constant  Value=100
  Integrator b{1..4} (4 alike) : DiscreteIntegrator  ExternalReset=either  InitialConditionSource=external  InitialCondition=510  InitialConditionSetting=State (most efficient)  SampleTime=-1
  MATLAB Function : MATLAB Function  Priority=1  TreatAsAtomicUnit=on
  MATLAB Function1 : MATLAB Function  TreatAsAtomicUnit=on
  Multiport Switch : MultiPortSwitch  Inputs=4
  Scope : Scope  NumInputPorts=8
      settings: TickLabels=on  ShowLegends=on  YMin=0~0~0~0~0~0~0~0  YMax=1~1~1~1~1~1~1~1
  q : Memory  X0=1  LinearizeMemory=on
  reset1 : Memory  LinearizeMemory=on
  xx : Memory  LinearizeMemory=on
  x : Outport
  wires:
  INIT y1/1 -> Integrator b1/3
  MATLAB Function1/1(ode1) -> Integrator b1/1
  MATLAB Function/1(qNext) -> q/1  "q_before"
  q/1 -> Multiport Switch/1, MATLAB Function/1(q), Scope/1  "q_after"
  MATLAB Function/2(reset) -> reset1/1
  MATLAB Function1/2(ode2) -> Integrator b2/1
  INIT y3/1 -> Integrator b3/3
  MATLAB Function1/3(ode3) -> Integrator b3/1
  MATLAB Function1/4(ode4) -> Integrator b4/1
  reset1/1 -> Integrator b4/2, Integrator b3/2, Integrator b2/2, Integrator b1/2  "reset_after"
  Integrator b1/1 -> Multiport Switch/2  "integrator t1"
  Integrator b2/1 -> Multiport Switch/3  "integrator t2"
  Integrator b3/1 -> Multiport Switch/4  "integrator t3"
  Integrator b4/1 -> Multiport Switch/5
  OFF/1 -> MATLAB Function/3(OFF)
  ON/1 -> MATLAB Function/2(ON)
  xx/1 -> x/1, Scope/2, Integrator b2/3, Integrator b4/3, MATLAB Function1/1(x), MATLAB Function/4(x)
  Multiport Switch/1 -> xx/1  "x"

== system waterTankBurner/waterTank48 ==
  note: integrator t4
  ON : Inport
  OFF : Inport  Port=2
  INIT y1 : Constant  Value=20
  INIT y3 : Constant  Value=100
  Integrator b{1..4} (4 alike) : DiscreteIntegrator  ExternalReset=either  InitialConditionSource=external  InitialCondition=510  InitialConditionSetting=State (most efficient)  SampleTime=-1
  MATLAB Function : MATLAB Function  Priority=1  TreatAsAtomicUnit=on
  MATLAB Function1 : MATLAB Function  TreatAsAtomicUnit=on
  Multiport Switch : MultiPortSwitch  Inputs=4
  Scope : Scope  NumInputPorts=8
      settings: TickLabels=on  ShowLegends=on  YMin=0~0~0~0~0~0~0~0  YMax=1~1~1~1~1~1~1~1
  q : Memory  X0=1  LinearizeMemory=on
  reset1 : Memory  LinearizeMemory=on
  xx : Memory  LinearizeMemory=on
  x : Outport
  wires:
  INIT y1/1 -> Integrator b1/3
  MATLAB Function1/1(ode1) -> Integrator b1/1
  MATLAB Function/1(qNext) -> q/1  "q_before"
  q/1 -> Multiport Switch/1, MATLAB Function/1(q), Scope/1  "q_after"
  MATLAB Function/2(reset) -> reset1/1
  MATLAB Function1/2(ode2) -> Integrator b2/1
  INIT y3/1 -> Integrator b3/3
  MATLAB Function1/3(ode3) -> Integrator b3/1
  MATLAB Function1/4(ode4) -> Integrator b4/1
  reset1/1 -> Integrator b4/2, Integrator b3/2, Integrator b2/2, Integrator b1/2  "reset_after"
  Integrator b1/1 -> Multiport Switch/2  "integrator t1"
  Integrator b2/1 -> Multiport Switch/3  "integrator t2"
  Integrator b3/1 -> Multiport Switch/4  "integrator t3"
  Integrator b4/1 -> Multiport Switch/5
  OFF/1 -> MATLAB Function/3(OFF)
  ON/1 -> MATLAB Function/2(ON)
  xx/1 -> x/1, Scope/2, Integrator b2/3, Integrator b4/3, MATLAB Function1/1(x), MATLAB Function/4(x)
  Multiport Switch/1 -> xx/1  "x"

== system waterTankBurner/waterTank49 ==
  note: integrator t4
  ON : Inport
  OFF : Inport  Port=2
  INIT y1 : Constant  Value=20
  INIT y3 : Constant  Value=100
  Integrator b{1..4} (4 alike) : DiscreteIntegrator  ExternalReset=either  InitialConditionSource=external  InitialCondition=510  InitialConditionSetting=State (most efficient)  SampleTime=-1
  MATLAB Function : MATLAB Function  Priority=1  TreatAsAtomicUnit=on
  MATLAB Function1 : MATLAB Function  TreatAsAtomicUnit=on
  Multiport Switch : MultiPortSwitch  Inputs=4
  Scope : Scope  NumInputPorts=8
      settings: TickLabels=on  ShowLegends=on  YMin=0~0~0~0~0~0~0~0  YMax=1~1~1~1~1~1~1~1
  q : Memory  X0=1  LinearizeMemory=on
  reset1 : Memory  LinearizeMemory=on
  xx : Memory  LinearizeMemory=on
  x : Outport
  wires:
  INIT y1/1 -> Integrator b1/3
  MATLAB Function1/1(ode1) -> Integrator b1/1
  MATLAB Function/1(qNext) -> q/1  "q_before"
  q/1 -> Multiport Switch/1, MATLAB Function/1(q), Scope/1  "q_after"
  MATLAB Function/2(reset) -> reset1/1
  MATLAB Function1/2(ode2) -> Integrator b2/1
  INIT y3/1 -> Integrator b3/3
  MATLAB Function1/3(ode3) -> Integrator b3/1
  MATLAB Function1/4(ode4) -> Integrator b4/1
  reset1/1 -> Integrator b4/2, Integrator b3/2, Integrator b2/2, Integrator b1/2  "reset_after"
  Integrator b1/1 -> Multiport Switch/2  "integrator t1"
  Integrator b2/1 -> Multiport Switch/3  "integrator t2"
  Integrator b3/1 -> Multiport Switch/4  "integrator t3"
  Integrator b4/1 -> Multiport Switch/5
  OFF/1 -> MATLAB Function/3(OFF)
  ON/1 -> MATLAB Function/2(ON)
  xx/1 -> x/1, Scope/2, Integrator b2/3, Integrator b4/3, MATLAB Function1/1(x), MATLAB Function/4(x)
  Multiport Switch/1 -> xx/1  "x"

== system waterTankBurner/waterTank5 ==
  note: integrator t4
  ON : Inport
  OFF : Inport  Port=2
  INIT y1 : Constant  Value=20
  INIT y3 : Constant  Value=100
  Integrator b{1..4} (4 alike) : DiscreteIntegrator  ExternalReset=either  InitialConditionSource=external  InitialCondition=510  InitialConditionSetting=State (most efficient)  SampleTime=-1
  MATLAB Function : MATLAB Function  Priority=1  TreatAsAtomicUnit=on
  MATLAB Function1 : MATLAB Function  TreatAsAtomicUnit=on
  Multiport Switch : MultiPortSwitch  Inputs=4
  Scope : Scope  NumInputPorts=8
      settings: TickLabels=on  ShowLegends=on  YMin=0~0~0~0~0~0~0~0  YMax=1~1~1~1~1~1~1~1
  q : Memory  X0=1  LinearizeMemory=on
  reset1 : Memory  LinearizeMemory=on
  xx : Memory  LinearizeMemory=on
  x : Outport
  wires:
  INIT y1/1 -> Integrator b1/3
  MATLAB Function1/1(ode1) -> Integrator b1/1
  MATLAB Function/1(qNext) -> q/1  "q_before"
  q/1 -> Multiport Switch/1, MATLAB Function/1(q), Scope/1  "q_after"
  MATLAB Function/2(reset) -> reset1/1
  MATLAB Function1/2(ode2) -> Integrator b2/1
  INIT y3/1 -> Integrator b3/3
  MATLAB Function1/3(ode3) -> Integrator b3/1
  MATLAB Function1/4(ode4) -> Integrator b4/1
  reset1/1 -> Integrator b4/2, Integrator b3/2, Integrator b2/2, Integrator b1/2  "reset_after"
  Integrator b1/1 -> Multiport Switch/2  "integrator t1"
  Integrator b2/1 -> Multiport Switch/3  "integrator t2"
  Integrator b3/1 -> Multiport Switch/4  "integrator t3"
  Integrator b4/1 -> Multiport Switch/5
  OFF/1 -> MATLAB Function/3(OFF)
  ON/1 -> MATLAB Function/2(ON)
  xx/1 -> x/1, Scope/2, Integrator b2/3, Integrator b4/3, MATLAB Function1/1(x), MATLAB Function/4(x)
  Multiport Switch/1 -> xx/1  "x"

== system waterTankBurner/waterTank6 ==
  note: integrator t4
  ON : Inport
  OFF : Inport  Port=2
  INIT y1 : Constant  Value=20
  INIT y3 : Constant  Value=100
  Integrator b{1..4} (4 alike) : DiscreteIntegrator  ExternalReset=either  InitialConditionSource=external  InitialCondition=510  InitialConditionSetting=State (most efficient)  SampleTime=-1
  MATLAB Function : MATLAB Function  Priority=1  TreatAsAtomicUnit=on
  MATLAB Function1 : MATLAB Function  TreatAsAtomicUnit=on
  Multiport Switch : MultiPortSwitch  Inputs=4
  Scope : Scope  NumInputPorts=8
      settings: TickLabels=on  ShowLegends=on  YMin=0~0~0~0~0~0~0~0  YMax=1~1~1~1~1~1~1~1
  q : Memory  X0=1  LinearizeMemory=on
  reset1 : Memory  LinearizeMemory=on
  xx : Memory  LinearizeMemory=on
  x : Outport
  wires:
  INIT y1/1 -> Integrator b1/3
  MATLAB Function1/1(ode1) -> Integrator b1/1
  MATLAB Function/1(qNext) -> q/1  "q_before"
  q/1 -> Multiport Switch/1, MATLAB Function/1(q), Scope/1  "q_after"
  MATLAB Function/2(reset) -> reset1/1
  MATLAB Function1/2(ode2) -> Integrator b2/1
  INIT y3/1 -> Integrator b3/3
  MATLAB Function1/3(ode3) -> Integrator b3/1
  MATLAB Function1/4(ode4) -> Integrator b4/1
  reset1/1 -> Integrator b4/2, Integrator b3/2, Integrator b2/2, Integrator b1/2  "reset_after"
  Integrator b1/1 -> Multiport Switch/2  "integrator t1"
  Integrator b2/1 -> Multiport Switch/3  "integrator t2"
  Integrator b3/1 -> Multiport Switch/4  "integrator t3"
  Integrator b4/1 -> Multiport Switch/5
  OFF/1 -> MATLAB Function/3(OFF)
  ON/1 -> MATLAB Function/2(ON)
  xx/1 -> x/1, Scope/2, Integrator b2/3, Integrator b4/3, MATLAB Function1/1(x), MATLAB Function/4(x)
  Multiport Switch/1 -> xx/1  "x"

== system waterTankBurner/waterTank7 ==
  note: integrator t4
  ON : Inport
  OFF : Inport  Port=2
  INIT y1 : Constant  Value=20
  INIT y3 : Constant  Value=100
  Integrator b{1..4} (4 alike) : DiscreteIntegrator  ExternalReset=either  InitialConditionSource=external  InitialCondition=510  InitialConditionSetting=State (most efficient)  SampleTime=-1
  MATLAB Function : MATLAB Function  Priority=1  TreatAsAtomicUnit=on
  MATLAB Function1 : MATLAB Function  TreatAsAtomicUnit=on
  Multiport Switch : MultiPortSwitch  Inputs=4
  Scope : Scope  NumInputPorts=8
      settings: TickLabels=on  ShowLegends=on  YMin=0~0~0~0~0~0~0~0  YMax=1~1~1~1~1~1~1~1
  q : Memory  X0=1  LinearizeMemory=on
  reset1 : Memory  LinearizeMemory=on
  xx : Memory  LinearizeMemory=on
  x : Outport
  wires:
  INIT y1/1 -> Integrator b1/3
  MATLAB Function1/1(ode1) -> Integrator b1/1
  MATLAB Function/1(qNext) -> q/1  "q_before"
  q/1 -> Multiport Switch/1, MATLAB Function/1(q), Scope/1  "q_after"
  MATLAB Function/2(reset) -> reset1/1
  MATLAB Function1/2(ode2) -> Integrator b2/1
  INIT y3/1 -> Integrator b3/3
  MATLAB Function1/3(ode3) -> Integrator b3/1
  MATLAB Function1/4(ode4) -> Integrator b4/1
  reset1/1 -> Integrator b4/2, Integrator b3/2, Integrator b2/2, Integrator b1/2  "reset_after"
  Integrator b1/1 -> Multiport Switch/2  "integrator t1"
  Integrator b2/1 -> Multiport Switch/3  "integrator t2"
  Integrator b3/1 -> Multiport Switch/4  "integrator t3"
  Integrator b4/1 -> Multiport Switch/5
  OFF/1 -> MATLAB Function/3(OFF)
  ON/1 -> MATLAB Function/2(ON)
  xx/1 -> x/1, Scope/2, Integrator b2/3, Integrator b4/3, MATLAB Function1/1(x), MATLAB Function/4(x)
  Multiport Switch/1 -> xx/1  "x"

== system waterTankBurner/waterTank8 ==
  note: integrator t4
  ON : Inport
  OFF : Inport  Port=2
  INIT y1 : Constant  Value=20
  INIT y3 : Constant  Value=100
  Integrator b{1..4} (4 alike) : DiscreteIntegrator  ExternalReset=either  InitialConditionSource=external  InitialCondition=510  InitialConditionSetting=State (most efficient)  SampleTime=-1
  MATLAB Function : MATLAB Function  Priority=1  TreatAsAtomicUnit=on
  MATLAB Function1 : MATLAB Function  TreatAsAtomicUnit=on
  Multiport Switch : MultiPortSwitch  Inputs=4
  Scope : Scope  NumInputPorts=8
      settings: TickLabels=on  ShowLegends=on  YMin=0~0~0~0~0~0~0~0  YMax=1~1~1~1~1~1~1~1
  q : Memory  X0=1  LinearizeMemory=on
  reset1 : Memory  LinearizeMemory=on
  xx : Memory  LinearizeMemory=on
  x : Outport
  wires:
  INIT y1/1 -> Integrator b1/3
  MATLAB Function1/1(ode1) -> Integrator b1/1
  MATLAB Function/1(qNext) -> q/1  "q_before"
  q/1 -> Multiport Switch/1, MATLAB Function/1(q), Scope/1  "q_after"
  MATLAB Function/2(reset) -> reset1/1
  MATLAB Function1/2(ode2) -> Integrator b2/1
  INIT y3/1 -> Integrator b3/3
  MATLAB Function1/3(ode3) -> Integrator b3/1
  MATLAB Function1/4(ode4) -> Integrator b4/1
  reset1/1 -> Integrator b4/2, Integrator b3/2, Integrator b2/2, Integrator b1/2  "reset_after"
  Integrator b1/1 -> Multiport Switch/2  "integrator t1"
  Integrator b2/1 -> Multiport Switch/3  "integrator t2"
  Integrator b3/1 -> Multiport Switch/4  "integrator t3"
  Integrator b4/1 -> Multiport Switch/5
  OFF/1 -> MATLAB Function/3(OFF)
  ON/1 -> MATLAB Function/2(ON)
  xx/1 -> x/1, Scope/2, Integrator b2/3, Integrator b4/3, MATLAB Function1/1(x), MATLAB Function/4(x)
  Multiport Switch/1 -> xx/1  "x"

== system waterTankBurner/waterTank9 ==
  note: integrator t4
  ON : Inport
  OFF : Inport  Port=2
  INIT y1 : Constant  Value=20
  INIT y3 : Constant  Value=100
  Integrator b{1..4} (4 alike) : DiscreteIntegrator  ExternalReset=either  InitialConditionSource=external  InitialCondition=510  InitialConditionSetting=State (most efficient)  SampleTime=-1
  MATLAB Function : MATLAB Function  Priority=1  TreatAsAtomicUnit=on
  MATLAB Function1 : MATLAB Function  TreatAsAtomicUnit=on
  Multiport Switch : MultiPortSwitch  Inputs=4
  Scope : Scope  NumInputPorts=8
      settings: TickLabels=on  ShowLegends=on  YMin=0~0~0~0~0~0~0~0  YMax=1~1~1~1~1~1~1~1
  q : Memory  X0=1  LinearizeMemory=on
  reset1 : Memory  LinearizeMemory=on
  xx : Memory  LinearizeMemory=on
  x : Outport
  wires:
  INIT y1/1 -> Integrator b1/3
  MATLAB Function1/1(ode1) -> Integrator b1/1
  MATLAB Function/1(qNext) -> q/1  "q_before"
  q/1 -> Multiport Switch/1, MATLAB Function/1(q), Scope/1  "q_after"
  MATLAB Function/2(reset) -> reset1/1
  MATLAB Function1/2(ode2) -> Integrator b2/1
  INIT y3/1 -> Integrator b3/3
  MATLAB Function1/3(ode3) -> Integrator b3/1
  MATLAB Function1/4(ode4) -> Integrator b4/1
  reset1/1 -> Integrator b4/2, Integrator b3/2, Integrator b2/2, Integrator b1/2  "reset_after"
  Integrator b1/1 -> Multiport Switch/2  "integrator t1"
  Integrator b2/1 -> Multiport Switch/3  "integrator t2"
  Integrator b3/1 -> Multiport Switch/4  "integrator t3"
  Integrator b4/1 -> Multiport Switch/5
  OFF/1 -> MATLAB Function/3(OFF)
  ON/1 -> MATLAB Function/2(ON)
  xx/1 -> x/1, Scope/2, Integrator b2/3, Integrator b4/3, MATLAB Function1/1(x), MATLAB Function/4(x)
  Multiport Switch/1 -> xx/1  "x"

== matlab function waterTankBurner/waterTank/MATLAB Function ==
  data: q input; ON input; OFF input; x input; qNext output; reset output


function [qNext,reset]  = phi(q,  ON, OFF,x)
%#codegen


if q==1 % q=1, tank is in t1
    if ON==0
        qNext=1;
        reset=0;
    elseif ON==1
        qNext=2;
        reset=1;
    else
        qNext=-1;
        reset=-1;
    end;
    
elseif q==2 % q=2, tank is in t2
    if x<100 && OFF==0
        qNext=2;
        reset=0;
    elseif x>=100
        qNext=3;
        reset=1;
    elseif x<100 && OFF==1
        qNext=4;
        reset=1;
    else
        qNext=-1;
        reset=-1;
    end;

elseif q==3 % q=3, tank is in state t3
    if OFF==0
        qNext=3;
        reset=0;
    elseif OFF==1
        qNext=4;
        reset=1;
    else
        qNext=-1;
        reset=-1;
    end;
elseif q==4 % q=4, tank is in state t4
    if x>20 && ON==0
        qNext=4;
        reset=0;
    elseif x<=20
        qNext=1;
        reset=1;
    elseif x>20 && ON==1
        qNext=2;
        reset=1;
    else
        qNext=-1;
        reset=-1;
    end;
else
    qNext=-1; %this should never execute
    reset=-1;%this should never execute
end

== matlab function waterTankBurner/Burner/MATLAB Function ==
  data: q input; TURN_ON input; TURN_OFF input; qNext output; ON output; OFF output; y input; reset output


function [qNext,ON,OFF,reset]  = phi(q,  TURN_ON, TURN_OFF,y)
%#codegen


if q==1 % q=1, burner is in state b1
    if TURN_ON==0
        qNext=1;
        reset=0;
        ON=0;
        OFF=0;
    elseif TURN_ON==1
        qNext=2;
        reset=1;
        ON=0;
        OFF=0;
    else
        qNext=-1;
        reset=-1;
        ON=-1;
        OFF=-1;
    end;
    
elseif q==2 % q=2, burner is in state b2
    if y>= 0.1
        qNext=3;
        reset=1;
        ON=1;
        OFF=0;
    elseif y< 0.1
        qNext=2;
        reset=0;
        ON=0;
        OFF=0;
    else
        qNext=-1;
        reset=-1;
        ON=-1;
        OFF=-1;
    end;

elseif q==3 % q=3, burner is in state b3
    if TURN_OFF==0
        qNext=3;
        reset=0;
        ON=0;
        OFF=0;
    elseif TURN_OFF==1
        qNext=4;
        reset=1;
        ON=0;
        OFF=0;
    else
        qNext=-1;
        reset=-1;
        ON=-1;
        OFF=-1;
    end;
elseif q==4 % q=4, burner is in state b4
    if y< 0.1
        qNext=4;
        reset=0;
        ON=0;
        OFF=0;
    elseif y>= 0.1
        qNext=1;
        reset=1;
        ON=0;
        OFF=1;
    else
        qNext=-1;
        reset=-1;
        ON=-1;
        OFF=-1;
    end;
else
    qNext=-1; %this should never execute
    reset=-1;%this should never execute
    ON=-1;%this should never execute
    OFF=-1;%this should never execute
    qNext=-1; %this should never execute
end

== matlab function waterTankBurner/waterTank/MATLAB Function1 ==
  data: x input; ode1 output; ode2 output; ode3 output; ode4 output
function [ode1,ode2,ode3,ode4] = ODEs(x)
%#codegen
K=0.075;
h=150;
ode1=0;
ode2=K*(h-x);
ode3=0;
ode4=-K*x;

== matlab function waterTankBurner/waterTank1/MATLAB Function ==
  data: q input; ON input; OFF input; x input; qNext output; reset output


function [qNext,reset]  = phi(q,  ON, OFF,x)
%#codegen


if q==1 % q=1, tank is in t1
    if ON==0
        qNext=1;
        reset=0;
    elseif ON==1
        qNext=2;
        reset=1;
    else
        qNext=-1;
        reset=-1;
    end;
    
elseif q==2 % q=2, tank is in t2
    if x<100 && OFF==0
        qNext=2;
        reset=0;
    elseif x>=100
        qNext=3;
        reset=1;
    elseif x<100 && OFF==1
        qNext=4;
        reset=1;
    else
        qNext=-1;
        reset=-1;
    end;

elseif q==3 % q=3, tank is in state t3
    if OFF==0
        qNext=3;
        reset=0;
    elseif OFF==1
        qNext=4;
        reset=1;
    else
        qNext=-1;
        reset=-1;
    end;
elseif q==4 % q=4, tank is in state t4
    if x>20 && ON==0
        qNext=4;
        reset=0;
    elseif x<=20
        qNext=1;
        reset=1;
    elseif x>20 && ON==1
        qNext=2;
        reset=1;
    else
        qNext=-1;
        reset=-1;
    end;
else
    qNext=-1; %this should never execute
    reset=-1;%this should never execute
end

== matlab function waterTankBurner/waterTank1/MATLAB Function1 ==
  data: x input; ode1 output; ode2 output; ode3 output; ode4 output
function [ode1,ode2,ode3,ode4] = ODEs(x)
%#codegen
K=0.075;
h=150;
ode1=0;
ode2=K*(h-x);
ode3=0;
ode4=-K*x;

== matlab function waterTankBurner/waterTank2/MATLAB Function ==
  data: q input; ON input; OFF input; x input; qNext output; reset output


function [qNext,reset]  = phi(q,  ON, OFF,x)
%#codegen


if q==1 % q=1, tank is in t1
    if ON==0
        qNext=1;
        reset=0;
    elseif ON==1
        qNext=2;
        reset=1;
    else
        qNext=-1;
        reset=-1;
    end;
    
elseif q==2 % q=2, tank is in t2
    if x<100 && OFF==0
        qNext=2;
        reset=0;
    elseif x>=100
        qNext=3;
        reset=1;
    elseif x<100 && OFF==1
        qNext=4;
        reset=1;
    else
        qNext=-1;
        reset=-1;
    end;

elseif q==3 % q=3, tank is in state t3
    if OFF==0
        qNext=3;
        reset=0;
    elseif OFF==1
        qNext=4;
        reset=1;
    else
        qNext=-1;
        reset=-1;
    end;
elseif q==4 % q=4, tank is in state t4
    if x>20 && ON==0
        qNext=4;
        reset=0;
    elseif x<=20
        qNext=1;
        reset=1;
    elseif x>20 && ON==1
        qNext=2;
        reset=1;
    else
        qNext=-1;
        reset=-1;
    end;
else
    qNext=-1; %this should never execute
    reset=-1;%this should never execute
end

== matlab function waterTankBurner/waterTank2/MATLAB Function1 ==
  data: x input; ode1 output; ode2 output; ode3 output; ode4 output
function [ode1,ode2,ode3,ode4] = ODEs(x)
%#codegen
K=0.075;
h=150;
ode1=0;
ode2=K*(h-x);
ode3=0;
ode4=-K*x;

== matlab function waterTankBurner/waterTank3/MATLAB Function ==
  data: q input; ON input; OFF input; x input; qNext output; reset output


function [qNext,reset]  = phi(q,  ON, OFF,x)
%#codegen


if q==1 % q=1, tank is in t1
    if ON==0
        qNext=1;
        reset=0;
    elseif ON==1
        qNext=2;
        reset=1;
    else
        qNext=-1;
        reset=-1;
    end;
    
elseif q==2 % q=2, tank is in t2
    if x<100 && OFF==0
        qNext=2;
        reset=0;
    elseif x>=100
        qNext=3;
        reset=1;
    elseif x<100 && OFF==1
        qNext=4;
        reset=1;
    else
        qNext=-1;
        reset=-1;
    end;

elseif q==3 % q=3, tank is in state t3
    if OFF==0
        qNext=3;
        reset=0;
    elseif OFF==1
        qNext=4;
        reset=1;
    else
        qNext=-1;
        reset=-1;
    end;
elseif q==4 % q=4, tank is in state t4
    if x>20 && ON==0
        qNext=4;
        reset=0;
    elseif x<=20
        qNext=1;
        reset=1;
    elseif x>20 && ON==1
        qNext=2;
        reset=1;
    else
        qNext=-1;
        reset=-1;
    end;
else
    qNext=-1; %this should never execute
    reset=-1;%this should never execute
end

== matlab function waterTankBurner/waterTank3/MATLAB Function1 ==
  data: x input; ode1 output; ode2 output; ode3 output; ode4 output
function [ode1,ode2,ode3,ode4] = ODEs(x)
%#codegen
K=0.075;
h=150;
ode1=0;
ode2=K*(h-x);
ode3=0;
ode4=-K*x;
